simulink model "Lab2_Second_Order"  (R2023a)
settings: Solver=ode4  StartTime=0.0  StopTime=15  FixedStep=1e-3  RelTol=1e-3
settings Model: Creator=Lenovo  LastModifiedBy=Lenovo

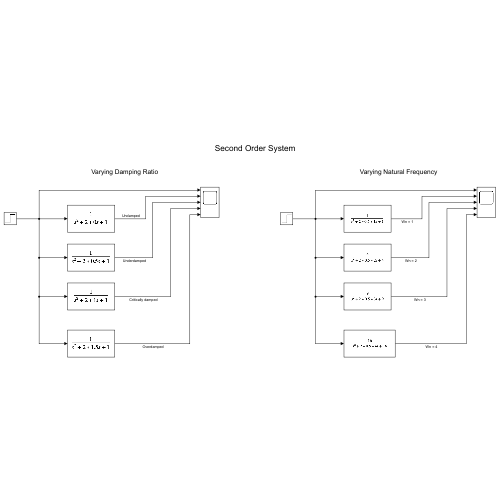
[thumbnail: Simulink's stored preview of the top-level diagram]
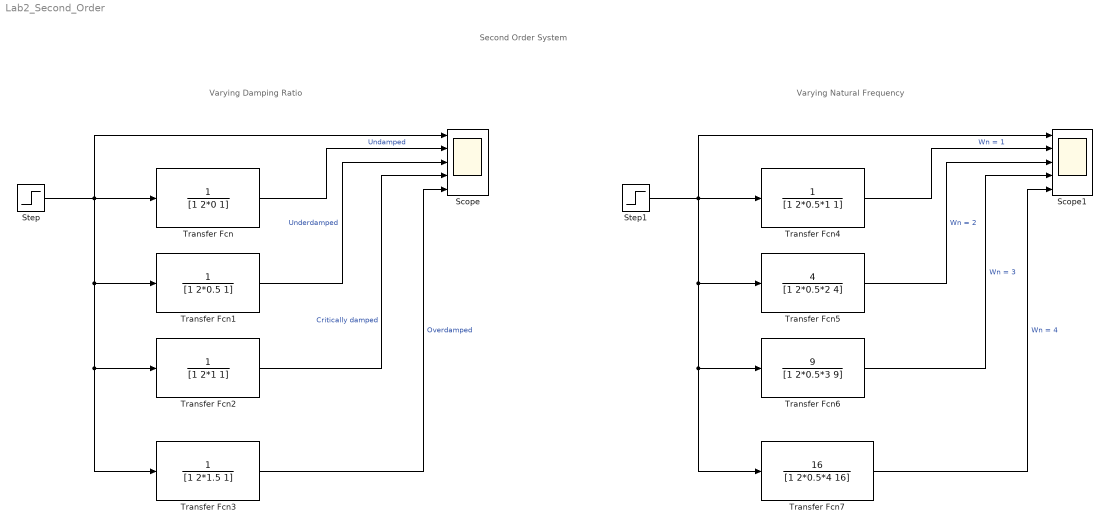
== system Lab2_Second_Order ==
  note: Second Order System
  note: Varying Damping Ratio
  note: Varying Natural Frequency
  Scope : Scope  NumInputPorts=5
  Scope1 : Scope  NumInputPorts=5
  Step : Step  SampleTime=0
  Step1 : Step  SampleTime=0
  Transfer Fcn : TransferFcn  Denominator=[1 2*0 1]
  Transfer Fcn1 : TransferFcn  Denominator=[1 2*0.5 1]
  Transfer Fcn2 : TransferFcn  Denominator=[1 2*1 1]
  Transfer Fcn3 : TransferFcn  Denominator=[1 2*1.5 1]
  Transfer Fcn4 : TransferFcn  Denominator=[1 2*0.5*1 1]
  Transfer Fcn5 : TransferFcn  Numerator=[4]  Denominator=[1 2*0.5*2 4]
  Transfer Fcn6 : TransferFcn  Numerator=[9]  Denominator=[1 2*0.5*3 9]
  Transfer Fcn7 : TransferFcn  Numerator=[16]  Denominator=[1 2*0.5*4 16]
  wires:
  Step/1 -> Transfer Fcn3/1, Transfer Fcn2/1, Transfer Fcn1/1, Scope/1, Transfer Fcn/1
  Transfer Fcn/1 -> Scope/2  "Undamped"
  Transfer Fcn1/1 -> Scope/3  "Underdamped"
  Transfer Fcn2/1 -> Scope/4  "Critically damped"
  Transfer Fcn3/1 -> Scope/5  "Overdamped"
  Transfer Fcn6/1 -> Scope1/4  "Wn = 3"
  Transfer Fcn7/1 -> Scope1/5  "Wn = 4"
  Step1/1 -> Transfer Fcn7/1, Transfer Fcn6/1, Transfer Fcn5/1, Scope1/1, Transfer Fcn4/1
  Transfer Fcn4/1 -> Scope1/2  "Wn = 1"
  Transfer Fcn5/1 -> Scope1/3  "Wn = 2"
